simulink model "balancingController_QP"  (Simulink 8.3)
settings: Solver=FixedStepDiscrete  StartTime=0.0  StopTime=simulationTime  FixedStep=Ts  RelTol=1e-3
InitFcn:
  | initBalancingController_QP;
values from neighbouring files (symbols this model uses):
  Aineq_f = [Aineq_fcone_f ... (first row only)    [initBalancingController_QP.m]
  bineq_f = [bineq_fcone_f ... (first row only)    [initBalancingController_QP.m]
  gains = [    120    0   1   1 ]    [initBalancingController_QP.m]
  impedances = [impTorso(1,:),impArms(1,:),impArms(1,:),impLegs(1,:),impLegs(1,:)]    [initBalancingControllerWithNonLinearImpedances.m]    (also in initBalancingController_QP.m)
  impedencesSat = [100   100    2000]    [initBalancingControllerWithNonLinearImpedances.m]    (also in initBalancingController_QP.m = [100   100    1000])
  increasingRatesImp = [impTorso(2,:),impArms(2,:),impArms(2,:),impLegs(2,:),impLegs(2,:)]    [initBalancingControllerWithNonLinearImpedances.m]    (also in initBalancingController_QP.m)
  referenceParams = [0.0 0.0]    [initBalancingControllerWithNonLinearImpedances.m]    (also in initBalancingController_QP.m)
  x0_lb_ub = block.InputPort(4).Data    [controllerQPsolver.m]    (also in initBalancingController_QP.m = [x0;lb;ub])
undefined symbols (not defined in the file or in its folder): DiscIntNeverNeededParam
libraries: WBCLibrary x20, simulink x2, dspsigops x2
settings Model: Creator=daniele  LastModifiedBy=talha
settings DataIOCC: SignalLoggingSaveFormat=Dataset
settings OptimizationCC: ExpressionDepthLimit=2147483647
settings DebuggingCC: FcnCallInpInsideContextMsg=EnableAllAsWarning
settings SFSimCC: SimParseCustomCode=off

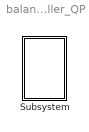
== system balancingController_QP ==
  Subsystem : Subsystem  mask{robotName='iCubGenova03', Ts=0.01, localName='balancingControllerQP'}
      mask prompts: robotName "robot name"; localName "module name"

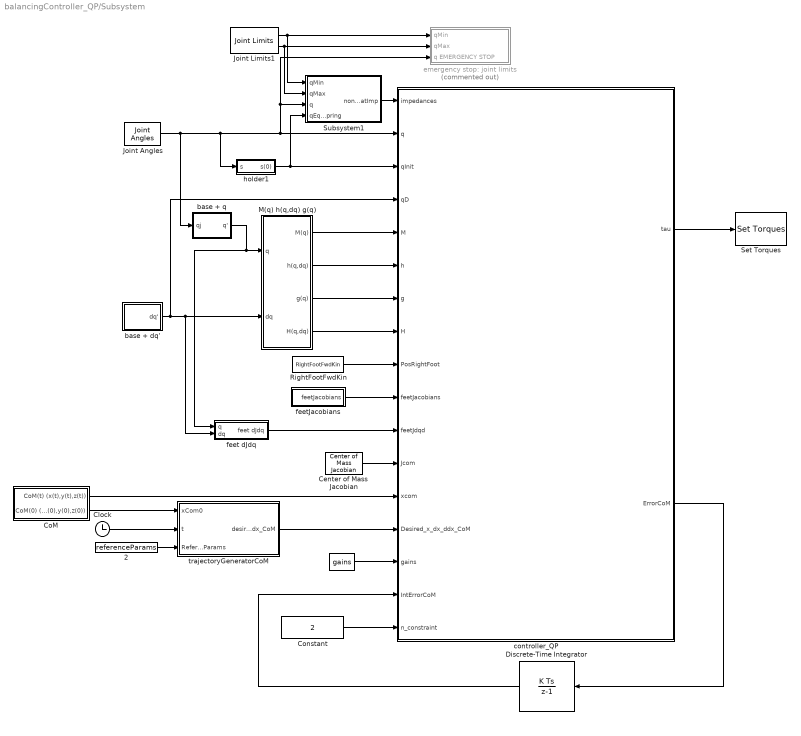
== system balancingController_QP/Subsystem ==
  "    " : Constant  Value=gains
  "    2" : Constant  Value=referenceParams
  Center of Mass Jacobian : WBCLibrary/wholeBodyModel/Jacobians/Center of Mass Jacobian  robotName=robotName  localName=localName
  Clock : Clock
  "CoM " : Subsystem
  Constant : Constant  Value=2
  Discrete-Time Integrator : DiscreteIntegrator  InitialCondition=[0 0 0]  SampleTime=Ts  ICPrevOutput=DiscIntNeverNeededParam  ICPrevScaledInput=DiscIntNeverNeededParam
  Joint Angles : WBCLibrary/wholeBodyStates/Joint Angles  robotName=robotName  localName=localName
  Joint Limits1 : WBCLibrary/wholeBodyModel/Joint Limits  robotName=robotName  localName=localName
  M(q) h(q,dq) g(q) : Subsystem
  RightFootFwdKin : WBCLibrary/wholeBodyModel/Forward Kinematics/RightFootFwdKin  robotName=robotName  localName=localName
  Set Torques : WBCLibrary/wholeBodyActuators/Set Torques  val=6  robotName=robotName  localName=localName
  Subsystem1 : Subsystem
  base + dq' : Subsystem
  base + q : Subsystem
  controller_QP : Subsystem
  emergency stop: joint limits : Subsystem  Commented=on
  feet dJdq : Subsystem
  feetJacobians : Subsystem
  holder1 : Subsystem
  trajectoryGeneratorCoM : MATLAB Function  TreatAsAtomicUnit=on
  wires:
  "    "/1 -> controller_QP/15(gains)
  trajectoryGeneratorCoM/1(desired_x_dx_ddx_CoM) -> controller_QP/14(Desired_x_dx_ddx_CoM)
  "CoM "/2(CoM(0) (x(0),y(0),z(0))) -> trajectoryGeneratorCoM/1(xCom0)
  RightFootFwdKin/1 -> controller_QP/9(PosRightFoot)
  Discrete-Time Integrator/1 -> controller_QP/16(IntErrorCoM)
  base + q/1(q') -> M(q) h(q,dq) g(q)/1(q), feet dJdq/1(q)
  Joint Angles/1 -> base + q/1(qj), Subsystem1/3(q), emergency stop: joint limits/3(q EMERGENCY STOP), controller_QP/2(q), holder1/1(s)
  M(q) h(q,dq) g(q)/3(g(q)) -> controller_QP/7(g)
  M(q) h(q,dq) g(q)/4(H(q,dq)) -> controller_QP/8(H)
  Center of Mass Jacobian/1 -> controller_QP/12(Jcom)
  feetJacobians/1(feetJacobians) -> controller_QP/10(feetJacobians)
  feet dJdq/1(feet dJdq) -> controller_QP/11(feetJdqd)
  holder1/1(s(0)) -> controller_QP/3(qInit), Subsystem1/4(qEquSpring)
  "CoM "/1(CoM(t) (x(t),y(t),z(t))) -> controller_QP/13(xcom)
  base + dq'/1(dq') -> controller_QP/4(qD), M(q) h(q,dq) g(q)/2(dq), feet dJdq/2(dq)
  M(q) h(q,dq) g(q)/1(M(q)) -> controller_QP/5(M)
  M(q) h(q,dq) g(q)/2(h(q,dq)) -> controller_QP/6(h)
  controller_QP/2(ErrorCoM) -> Discrete-Time Integrator/1
  Constant/1 -> controller_QP/17(n_constraint)
  controller_QP/1(tau) -> Set Torques/1
  "    2"/1 -> trajectoryGeneratorCoM/3(ReferenceParams)
  Clock/1 -> trajectoryGeneratorCoM/2(t)
  Subsystem1/1(nonLinSatImp) -> controller_QP/1(impedances)
  Joint Limits1/1 -> emergency stop: joint limits/1(qMin), Subsystem1/1(qMin)
  Joint Limits1/2 -> emergency stop: joint limits/2(qMax), Subsystem1/2(qMax)

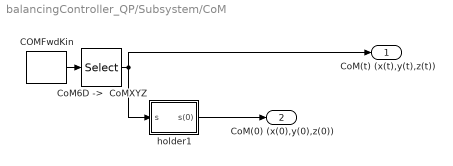
== system balancingController_QP/Subsystem/CoM  ==
  "COMFwdKin " : WBCLibrary/wholeBodyModel/Forward Kinematics/COMFwdKin   robotName=robotName  localName=localName
  "CoM6D ->  CoMXYZ" : Selector  InputPortWidth=7  Indices=[1 2 3]
  holder1 : Subsystem
  CoM(t) (x(t),y(t),z(t)) : Outport
  CoM(0) (x(0),y(0),z(0)) : Outport  Port=2
  wires:
  "COMFwdKin "/1 -> "CoM6D ->  CoMXYZ"/1
  "CoM6D ->  CoMXYZ"/1 -> holder1/1(s), CoM(t) (x(t),y(t),z(t))/1
  holder1/1(s(0)) -> CoM(0) (x(0),y(0),z(0))/1

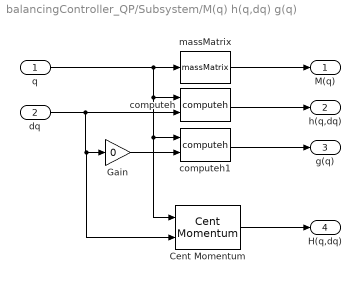
== system balancingController_QP/Subsystem/M(q) h(q,dq) g(q) ==
  q : Inport
  dq : Inport  Port=2
  Cent Momentum : WBCLibrary/wholeBodyModel/Dynamics/Cent Momentum  robotName=robotName  localName=localName
  Gain : Gain  Gain=0
  computeh : WBCLibrary/wholeBodyModel/Dynamics/computeh  val=7  robotname=robotName  localname=localName
  computeh1 : WBCLibrary/wholeBodyModel/Dynamics/computeh  val=7  robotname=robotName  localname=localName
  massMatrix : WBCLibrary/wholeBodyModel/Dynamics/massMatrix  val=8  robotname=robotName  localname=localName
  M(q) : Outport
  h(q,dq) : Outport  Port=2
  g(q) : Outport  Port=3
  H(q,dq) : Outport  Port=4
  wires:
  Gain/1 -> computeh1/2
  computeh1/1 -> g(q)/1
  computeh/1 -> h(q,dq)/1
  massMatrix/1 -> M(q)/1
  q/1 -> Cent Momentum/1, computeh1/1, computeh/1, massMatrix/1
  dq/1 -> Cent Momentum/2, Gain/1, computeh/2
  Cent Momentum/1 -> H(q,dq)/1

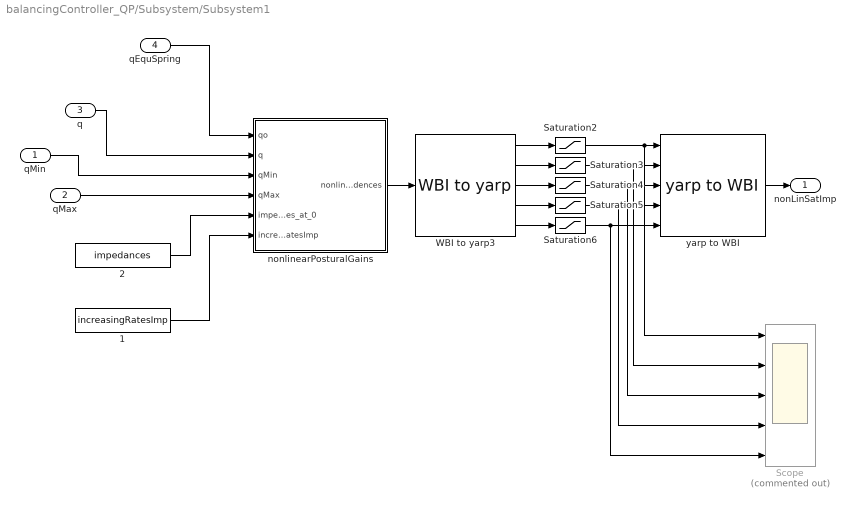
== system balancingController_QP/Subsystem/Subsystem1 ==
  qMin : Inport
  qMax : Inport  Port=2
  q : Inport  Port=3
  qEquSpring : Inport  Port=4
  "    1" : Constant  Value=increasingRatesImp
  "    2" : Constant  Value=impedances
  Saturation2 : Saturate  UpperLimit=impedencesSat(1)  LowerLimit=0  SampleTime=Ts
  Saturation3 : Saturate  UpperLimit=impedencesSat(2)  LowerLimit=0  SampleTime=Ts
  Saturation4 : Saturate  UpperLimit=impedencesSat(2)  LowerLimit=0  SampleTime=Ts
  Saturation5 : Saturate  UpperLimit=impedencesSat(3)  LowerLimit=0  SampleTime=Ts
  Saturation6 : Saturate  UpperLimit=impedencesSat(3)  LowerLimit=0  SampleTime=Ts
  Scope : Scope  Commented=on  NumInputPorts=5
      settings: ShowLegends=on  TimeRange=12  YMin=-5~-5~-5~0.9370629370629331~-5  YMax=5~5~5~4.937062937062933~5
  WBI to yarp3 : WBCLibrary/Utilities/WBI to yarp
  "nonlinearPosturalGains " : MATLAB Function  TreatAsAtomicUnit=on
  yarp to WBI : WBCLibrary/Utilities/yarp to WBI
  nonLinSatImp : Outport
  wires:
  WBI to yarp3/1 -> Saturation2/1
  WBI to yarp3/2 -> Saturation3/1
  WBI to yarp3/3 -> Saturation4/1
  WBI to yarp3/4 -> Saturation5/1
  WBI to yarp3/5 -> Saturation6/1
  "nonlinearPosturalGains "/1(nonlinearImpedences) -> WBI to yarp3/1
  yarp to WBI/1 -> nonLinSatImp/1
  qEquSpring/1 -> "nonlinearPosturalGains "/1(qo)
  qMin/1 -> "nonlinearPosturalGains "/3(qMin)
  qMax/1 -> "nonlinearPosturalGains "/4(qMax)
  "    2"/1 -> "nonlinearPosturalGains "/5(impedences_at_0)
  "    1"/1 -> "nonlinearPosturalGains "/6(increasingRatesImp)
  q/1 -> "nonlinearPosturalGains "/2(q)
  Saturation6/1 -> Scope/5, yarp to WBI/5
  Saturation4/1 -> Scope/3, yarp to WBI/3
  Saturation5/1 -> Scope/4, yarp to WBI/4
  Saturation3/1 -> Scope/2, yarp to WBI/2
  Saturation2/1 -> Scope/1, yarp to WBI/1

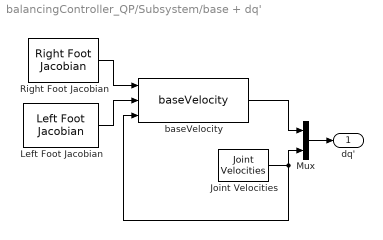
== system balancingController_QP/Subsystem/base + dq' ==
  Joint Velocities : WBCLibrary/wholeBodyStates/Joint Velocities  robotName=robotName  localName=localName
  Left Foot Jacobian : WBCLibrary/wholeBodyModel/Jacobians/Left Foot Jacobian  robotName=robotName  localName=localName
  Mux : Mux  Inputs=2
  Right Foot Jacobian : WBCLibrary/wholeBodyModel/Jacobians/Right Foot Jacobian  robotName=robotName  localName=localName
  baseVelocity : WBCLibrary/Utilities/baseVelocity
  dq' : Outport
  wires:
  Left Foot Jacobian/1 -> baseVelocity/2
  Right Foot Jacobian/1 -> baseVelocity/1
  baseVelocity/1 -> Mux/1
  Joint Velocities/1 -> baseVelocity/3, Mux/2
  Mux/1 -> dq'/1

== system balancingController_QP/Subsystem/base + q ==
  qj : Inport
  Constant1 : Constant  Value=zeros(16,1)
  Mux : Mux  Inputs=2
  q' : Outport
  wires:
  Mux/1 -> q'/1
  qj/1 -> Mux/2
  Constant1/1 -> Mux/1

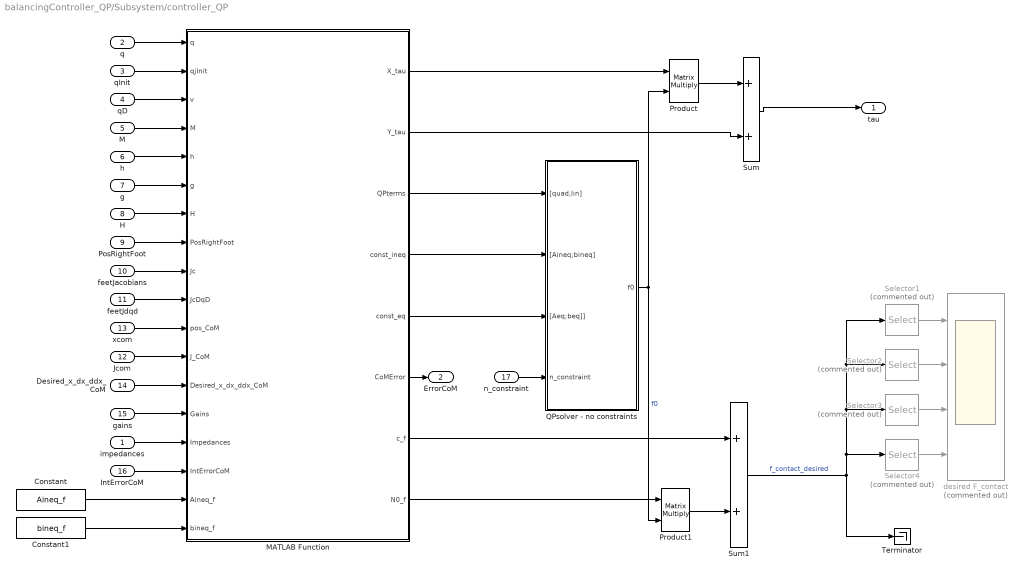
== system balancingController_QP/Subsystem/controller_QP ==
  impedances : Inport
  q : Inport  Port=2
  qInit : Inport  Port=3
  qD : Inport  Port=4
  M : Inport  Port=5
  h : Inport  Port=6
  g : Inport  Port=7
  H : Inport  Port=8
  PosRightFoot : Inport  Port=9
  feetJacobians : Inport  Port=10
  feetJdqd : Inport  Port=11
  Jcom : Inport  Port=12
  xcom : Inport  Port=13
  Desired_x_dx_ddx_CoM : Inport  Port=14
  gains : Inport  Port=15
  IntErrorCoM : Inport  Port=16
  n_constraint : Inport  Port=17
  Constant : Constant  Value=Aineq_f
  Constant1 : Constant  Value=bineq_f
  MATLAB Function : MATLAB Function  TreatAsAtomicUnit=on
  Product : Product  Multiplication=Matrix(*)
  Product1 : Product  Multiplication=Matrix(*)
  QPsolver - no constraints : Subsystem
  Selector1 : Selector  Commented=on  InputPortWidth=12  Indices=[1 2 3]
  Selector2 : Selector  Commented=on  InputPortWidth=12  Indices=[4 5 6]
  Selector3 : Selector  Commented=on  InputPortWidth=12  Indices=[7 8 9]
  Selector4 : Selector  Commented=on  InputPortWidth=12  Indices=[10 11 12]
  Sum : Sum
  Sum1 : Sum
  Terminator : Terminator
  desired F_contact : Scope  Commented=on  NumInputPorts=4
      settings: YMin=-5~-5~-5~-5  YMax=5~5~5~5  SaveName=ScopeData2
  tau : Outport
  ErrorCoM : Outport  Port=2
  wires:
  q/1 -> MATLAB Function/1(q)
  qInit/1 -> MATLAB Function/2(qjInit)
  qD/1 -> MATLAB Function/3(v)
  M/1 -> MATLAB Function/4(M)
  h/1 -> MATLAB Function/5(h)
  g/1 -> MATLAB Function/6(g)
  H/1 -> MATLAB Function/7(H)
  PosRightFoot/1 -> MATLAB Function/8(PosRightFoot)
  feetJacobians/1 -> MATLAB Function/9(Jc)
  feetJdqd/1 -> MATLAB Function/10(JcDqD)
  xcom/1 -> MATLAB Function/11(pos_CoM)
  Jcom/1 -> MATLAB Function/12(J_CoM)
  Desired_x_dx_ddx_CoM/1 -> MATLAB Function/13(Desired_x_dx_ddx_CoM)
  gains/1 -> MATLAB Function/14(Gains)
  impedances/1 -> MATLAB Function/15(Impedances)
  IntErrorCoM/1 -> MATLAB Function/16(IntErrorCoM)
  n_constraint/1 -> QPsolver - no constraints/4(n_constraint)
  MATLAB Function/6(CoMError) -> ErrorCoM/1
  MATLAB Function/3(QPterms) -> QPsolver - no constraints/1("[quad,lin]")
  MATLAB Function/4(const_ineq) -> QPsolver - no constraints/2("[Aineq;bineq]")
  MATLAB Function/5(const_eq) -> QPsolver - no constraints/3("[Aeq;beq]]")
  QPsolver - no constraints/1(f0) -> Product1/2, Product/2  "f0"
  Product/1 -> Sum/1
  Sum/1 -> tau/1
  MATLAB Function/1(X_tau) -> Product/1
  MATLAB Function/2(Y_tau) -> Sum/2
  MATLAB Function/8(N0_f) -> Product1/1
  Product1/1 -> Sum1/2
  MATLAB Function/7(c_f) -> Sum1/1
  Sum1/1 -> Selector4/1, Selector3/1, Selector2/1, Selector1/1, Terminator/1  "f_contact_desired"
  Selector1/1 -> desired F_contact/1
  Selector4/1 -> desired F_contact/4
  Selector3/1 -> desired F_contact/3
  Selector2/1 -> desired F_contact/2
  Constant/1 -> MATLAB Function/17(Aineq_f)
  Constant1/1 -> MATLAB Function/18(bineq_f)

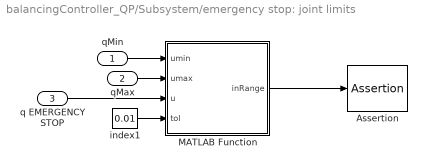
== system balancingController_QP/Subsystem/emergency stop: joint limits ==
  qMin : Inport
  qMax : Inport  Port=2
  q EMERGENCY STOP : Inport  Port=3
  Assertion : Assertion
  MATLAB Function : MATLAB Function  TreatAsAtomicUnit=on
  index1 : Constant  Value=0.01  VectorParams1D=off
  wires:
  qMin/1 -> MATLAB Function/1(umin)
  qMax/1 -> MATLAB Function/2(umax)
  index1/1 -> MATLAB Function/4(tol)
  q EMERGENCY STOP/1 -> MATLAB Function/3(u)
  MATLAB Function/1(inRange) -> Assertion/1

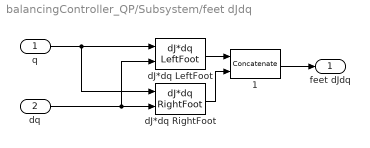
== system balancingController_QP/Subsystem/feet dJdq ==
  q : Inport
  dq : Inport  Port=2
  " 1" : Concatenate  Mode=Multidimensional array
  dJ*dq LeftFoot : WBCLibrary/wholeBodyModel/Dynamics/dJ*dq LeftFoot  val=9  robotName=robotName  localName=localName
  dJ*dq RightFoot : WBCLibrary/wholeBodyModel/Dynamics/dJ*dq RightFoot  val=9  robotName=robotName  localName=localName
  feet dJdq : Outport
  wires:
  dJ*dq LeftFoot/1 -> " 1"/1
  dJ*dq RightFoot/1 -> " 1"/2
  " 1"/1 -> feet dJdq/1
  q/1 -> dJ*dq RightFoot/1, dJ*dq LeftFoot/1
  dq/1 -> dJ*dq LeftFoot/2, dJ*dq RightFoot/2

== system balancingController_QP/Subsystem/feetJacobians ==
  " " : Concatenate  Mode=Multidimensional array
  Left Foot Jacobian : WBCLibrary/wholeBodyModel/Jacobians/Left Foot Jacobian  robotName=robotName  localName=localName
  Right Foot Jacobian : WBCLibrary/wholeBodyModel/Jacobians/Right Foot Jacobian  robotName=robotName  localName=localName
  feetJacobians : Outport
  wires:
  Left Foot Jacobian/1 -> " "/1
  Right Foot Jacobian/1 -> " "/2
  " "/1 -> feetJacobians/1

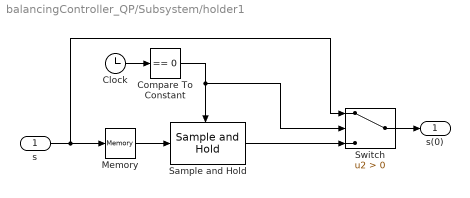
== system balancingController_QP/Subsystem/holder1 ==
  s : Inport
  Clock : Clock
  Compare To Constant : simulink/Logic and Bit Operations/Compare To Constant  relop===  const=0  OutDataTypeStr=boolean
  Memory : Memory
  Sample and Hold : dspsigops/Sample and Hold  trig=Falling edge  initCond=0  latchinput=off
  Switch : Switch  Criteria=u2 > Threshold
  s(0) : Outport
  wires:
  s/1 -> Switch/1, Memory/1
  Clock/1 -> Compare To Constant/1
  Compare To Constant/1 -> Sample and Hold/Trigger, Switch/2
  Sample and Hold/1 -> Switch/3
  Switch/1 -> s(0)/1
  Memory/1 -> Sample and Hold/1

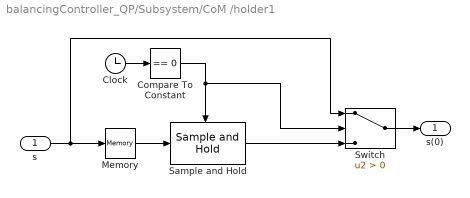
== system balancingController_QP/Subsystem/CoM /holder1 ==
  s : Inport
  Clock : Clock
  Compare To Constant : simulink/Logic and Bit Operations/Compare To Constant  relop===  const=0  OutDataTypeStr=boolean
  Memory : Memory
  Sample and Hold : dspsigops/Sample and Hold  trig=Falling edge  initCond=0  latchinput=off
  Switch : Switch  Criteria=u2 > Threshold
  s(0) : Outport
  wires:
  s/1 -> Switch/1, Memory/1
  Clock/1 -> Compare To Constant/1
  Compare To Constant/1 -> Sample and Hold/Trigger, Switch/2
  Sample and Hold/1 -> Switch/3
  Switch/1 -> s(0)/1
  Memory/1 -> Sample and Hold/1

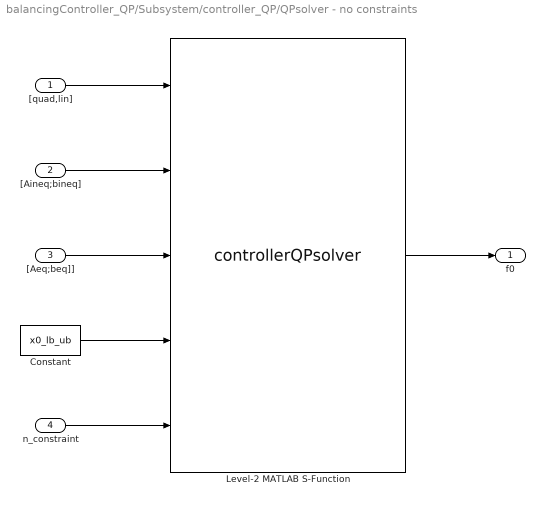
== system balancingController_QP/Subsystem/controller_QP/QPsolver - no constraints ==
  "[quad,lin]" : Inport
  "[Aineq;bineq]" : Inport  Port=2
  "[Aeq;beq]]" : Inport  Port=3
  n_constraint : Inport  Port=4
  Constant : Constant  Value=x0_lb_ub
  Level-2 MATLAB S-Function : M-S-Function  FunctionName=controllerQPsolver
  f0 : Outport
  wires:
  "[quad,lin]"/1 -> Level-2 MATLAB S-Function/1
  "[Aineq;bineq]"/1 -> Level-2 MATLAB S-Function/2
  "[Aeq;beq]]"/1 -> Level-2 MATLAB S-Function/3
  Constant/1 -> Level-2 MATLAB S-Function/4
  Level-2 MATLAB S-Function/1 -> f0/1
  n_constraint/1 -> Level-2 MATLAB S-Function/5

== matlab function Subsystem/trajectoryGeneratorCoM ==
  data: desired_x_dx_ddx_CoM output double; xCom0 input double; t input double; ReferenceParams input double
function desired_x_dx_ddx_CoM = fcn(xCom0,t,ReferenceParams)
%#codegen

e3 = [0;1;0];
A = ReferenceParams(1);
f = ReferenceParams(2);

xcomDes    = xCom0 + A*sin(2*pi*f*t)*e3;
% xcomDes(1) =  xcomDes(1) + 0.01;
xDcomDes   =         A*2*pi*f*cos(2*pi*f*t)*e3;
xDDcomDes  =        -A*(2*pi*f)^2*sin(2*pi*f*t)*e3;

desired_x_dx_ddx_CoM = [xcomDes,xDcomDes,xDDcomDes];

== matlab function Subsystem/controller_QP/MATLAB Function ==
  data: q input double; X_tau output double; Y_tau output double; QPterms output double; const_ineq output double; const_eq output double; qjInit input double; v input double; M input double; h input double; g input double; H input double; PosRightFoot input double; Jc input double; JcDqD input double; pos_CoM input double; J_CoM input double; Desired_x_dx_ddx_CoM input double; Gains input double; Impedances input double; IntErrorCoM input double; CoMError output double; c_f output double; N0_f output double; Aineq_f input double; bineq_f input double
function [X_tau,Y_tau,QPterms,const_ineq,const_eq,CoMError,c_f,N0_f]  =  fcnQP_part1(q,qjInit,v, M, h, g, H, PosRightFoot, Jc, JcDqD, pos_CoM,J_CoM, Desired_x_dx_ddx_CoM, Gains, Impedances, IntErrorCoM,Aineq_f,bineq_f)
   
n_constraint    = 2;
n_dof           = 25;
PINV_TOL        = 1e-5;
gravAcc         = 9.81;
m               = M(1,1);
Mb              = M(1:6,1:6);
Mbj             = M(1:6,7:end);

St              = [  zeros(6,n_dof);
                   eye(n_dof,n_dof)];
grav            = [ zeros(2,1);
                   -m*gravAcc;
                    zeros(3,1)];
pos_rightFoot   = PosRightFoot(1:3);
JcMinv          = Jc/M;
JcMinvSt        = JcMinv*St;
JcMinvJct       = JcMinv*transpose(Jc);
xDcom           = J_CoM(1:3,:)*v;
xDDcomStar      = Desired_x_dx_ddx_CoM(:,3) - Gains(1)*(pos_CoM - Desired_x_dx_ddx_CoM(:,1)) - Gains(2)*IntErrorCoM - Gains(3)*(xDcom - Desired_x_dx_ddx_CoM(:,2));
Pr              =  pos_rightFoot - pos_CoM; % Application point of the contact force on the right foot w.r.t. CoM

switch n_constraint
    case 1 % on left foot
        A  = [ eye(3),   zeros(3);
             -Sf(pos_CoM),  eye(3)];
    case 2 % on both feet
        A  = [ eye(3),   zeros(3),eye(3), zeros(3);
             -Sf(pos_CoM),  eye(3), Sf(Pr), eye(3) ];
    otherwise
        disp('Choose number of constraints properly (1 or 2)');
        return
end        

pinvA         = pinv(        A, PINV_TOL);
PInv_JcMinvSt = pinv( JcMinvSt, PINV_TOL);
HDotDes       = [    m*xDDcomStar ;
                -Gains(4)*H(4:end)]; 
         
%% QP FOR TORQUE MINIMIZATION BASED ON arbitrary vector F0

%define tau_0 (the arbitrary vector)
mult_f_tau0   =  Mbj'/Mb*transpose(Jc(:,1:6))-transpose(Jc(:,7:end)); % multiplier of f in tau0
n_tau0        =  g(7:end) - Impedances.*(q-qjInit) - Mbj'/Mb*h(1:6); % additional terms in tau0
%

N0_tau        = eye(n_dof) - PInv_JcMinvSt*JcMinvSt;
mult_f_tau    = PInv_JcMinvSt*(-JcMinvJct)+N0_tau*mult_f_tau0;
n_tau         = PInv_JcMinvSt*(JcMinv*h-JcDqD)+N0_tau*n_tau0;

% f desired is given as:
% f*   = pinvA*(HDotDes - grav)  + (I-pinvA*A) * f0
% f*   =           c_f           +     N0_f    * f0
N0_f          = eye(6*n_constraint,6*n_constraint)-pinvA*A;
c_f           = pinvA*(HDotDes - grav);

% tau is given as:
% tau = (mult_f_tau*N0_f)* f0 + (n_tau+mult_f_tau*c_f)
% tau =        X_tau     * f0 +                   Y_tau

X_tau         = mult_f_tau*N0_f;
Y_tau         = n_tau + mult_f_tau*c_f;
quadraticTerm = 2*(transpose(X_tau)*X_tau)+eye(6*n_constraint)*1e-8;
linearTerm    = transpose(2*X_tau'*Y_tau);

% rewrite constraints in terms of f0
Aineq = Aineq_f*N0_f;
bineq = bineq_f-Aineq_f*c_f;

Aeq = zeros(1,12);
beq = zeros(1,1);

QPterms     = reshape([quadraticTerm;linearTerm],1,[]);
const_ineq  = reshape([Aineq,bineq],1,[]);
const_eq    = reshape([Aeq,beq],1,[]);
CoMError    = pos_CoM - Desired_x_dx_ddx_CoM(:,1);

== matlab function Subsystem/emergency stop: joint limits/MATLAB Function ==
  data: umin input double; umax input double; u input double; inRange output double; tol input double
function inRange = checkRange(umin, umax, u, tol)
%#codegen

res = u < umin + tol | u > umax - tol;
res = sum(res);
if res==0
    inRange = 1;
else
    inRange = 0;
    u < umin + tol | u > umax - tol
end

== matlab function Subsystem/Subsystem1/nonlinearPosturalGains  ==
  data: qo input double; nonlinearImpedences output double; q input double; qMin input double; qMax input double; impedences_at_0 input double; increasingRatesImp input double
function nonlinearImpedences = fcn(qo,q,qMin,qMax,impedences_at_0,increasingRatesImp)
    %#codegen

    tp =  pi./(2*(qMax-qo));
    tn = -pi./(2*(qMin-qo));

    qTilde = q - qo;
            
    nonlinearImpedences = impedences_at_0' + (increasingRatesImp.*tan((tp.*stepFcn(qTilde) + tn.*stepFcn(-qTilde)).*qTilde).^2)' ;
end

function y = stepFcn(x) 
   %#codegen
   y = x > 0; 
end
